simulink model "EXAMPLE_EncodeMavlink_blocks"  (R2019b)
settings: Solver=FixedStepAuto  StartTime=0.0  StopTime=inf  FixedStep=0.01  RelTol=1e-3  EnableMultiTasking=on
libraries: commutil2 x10, etargetslib x10, simulink x9, commcrc2 x5, px4uORBlib x2, px4Sensorslib x2, px4lib x1
settings Model: SimulationMode=external  ExtModeTrigDuration=10  Creator=Admin  LastModifiedBy=andrei
settings SolverCC: PositivePriorityOrder=on
settings DataIOCC: ReturnWorkspaceOutputs=off
settings OptimizationCC: EnhancedBackFolding=on  PassReuseOutputArgsAs=Individual arguments  MaxStackSize=64  OptimizeBlockOrder=speed  DifferentSizesBufferReuse=on  OptimizationCustomize=off  EfficientTunableParamExpr=on
settings DebuggingCC: ParameterTunabilityLossMsg=error  ArithmeticOperatorsInVariantConditions=warning
settings HardwareCC: ProdBitPerPointer=32  ProdBitPerSizeT=32  ProdBitPerPtrDiffT=32  ProdLargestAtomicInteger=Long  ProdLargestAtomicFloat=Double  ProdWordSize=32  ProdLongLongMode=on  ProdHWDeviceType=ARM Compatible->ARM Cortex
settings SFSimCC: SimUseLocalCustomCode=off  MATLABDynamicMemAlloc=off  CustomCodeUndefinedFunction=UseInterfaceOnly
settings RTWCC: SystemTargetFile=ert.tlc  HardwareBoard=PX4 Pixhawk 1  TLCOptions="-aInlineSetEventsForThisBaseRateFcn=TLC_FALSE -aSuppressMultiTaskScheduler=TLC_FALSE  -aRateBasedStepFcn=0"  TemplateMakefile=ert_default_tmf  GenerateReport=on  RTWUseLocalCustomCode=off  Toolchain=GNU Tools for PX4 Autopilots  IncludeHyperlinkInReport=on  LaunchReport=on  TargetLang=C++  GenerateTraceInfo=on  GenerateTraceReport=on  GenerateTraceReportSl=on  GenerateTraceReportSf=on  GenerateTraceReportEml=on
settings CodeAppCC: ForceParamTrailComments=on  IgnoreCustomStorageClasses=off  OperatorAnnotations=on  SimulinkDataObjDesc=on  SFDataObjDesc=on  InsertBlockDesc=on
settings ERTTargetCC: SupportNonInlinedSFcns=on

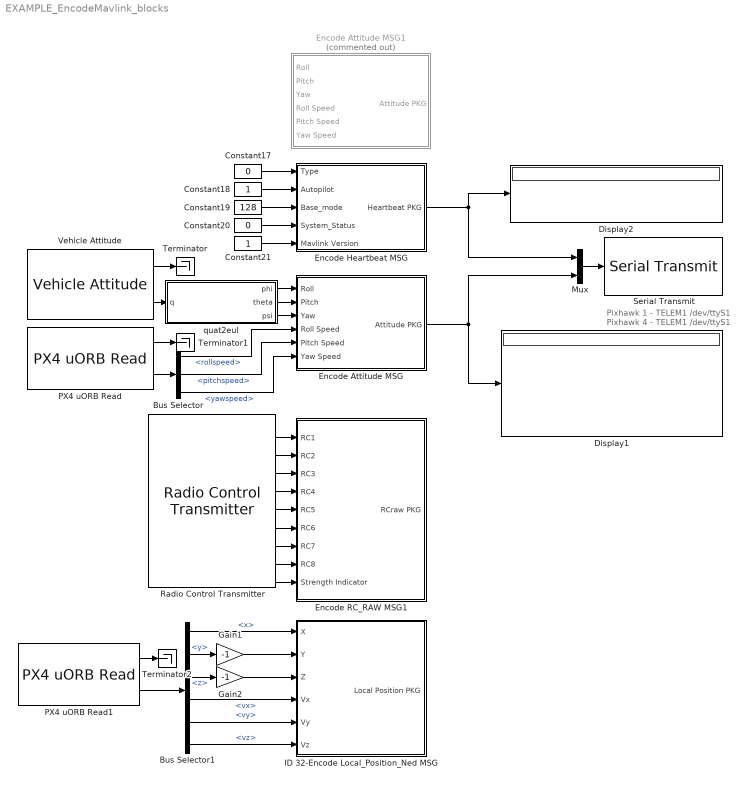
== system EXAMPLE_EncodeMavlink_blocks ==
  note: Pixhawk 1 - TELEM1 /dev/ttyS1
      | Pixhawk 4 - TELEM1 /dev/ttyS1
  Bus Selector : BusSelector  OutputSignals=rollspeed,pitchspeed,yawspeed
  Bus Selector1 : BusSelector  OutputSignals=x,y,z,vx,vy,vz
  Constant17 : Constant  Value=0
  Constant18 : Constant
  Constant19 : Constant  Value=128
  Constant20 : Constant  Value=0
  Constant21 : Constant
  Display1 : Display
  Display2 : Display
  Encode Attitude MSG : Subsystem
  Encode Attitude MSG1 : Subsystem  Commented=on
  Encode Heartbeat MSG : Subsystem
  Encode RC_RAW MSG1 : Subsystem
  Gain1 : Gain  Gain=-1
  Gain2 : Gain  Gain=-1
  ID 32-Encode Local_Position_Ned MSG : Subsystem
  Mux : Mux  Inputs=2
  PX4 uORB Read : px4uORBlib/PX4 uORB Read  uORBTopic=vehicle_attitude  sampleTime=0.01  BlockingMode=off  BlockTimeout=1e-3
      settings: SourceProductName=Embedded Coder Support Package for PX4 Autopilots  SourceProductBaseCode=PX4AUTOPILOTS
  PX4 uORB Read1 : px4uORBlib/PX4 uORB Read  uORBTopic=vehicle_local_position  sampleTime=0.01  BlockingMode=off  BlockTimeout=1e-3
      settings: SourceProductName=Embedded Coder Support Package for PX4 Autopilots  SourceProductBaseCode=PX4AUTOPILOTS
  Radio Control Transmitter : px4Sensorslib/Radio Control Transmitter  channel1=on  channel2=on  channel3=on  channel4=on  channel5=on  channel6=on  channel7=on  channel8=on  channel_count=off  rssi=on  rc_input_source=off  timestamp_last_signal=off  time_stamp=off  sampleTime=1/250  BlockingMode=off  BlockTimeout=5
      settings: SourceProductName=Embedded Coder Support Package for PX4 Autopilots
  Serial Transmit : px4lib/Serial Transmit  SCIModule=/dev/ttyS1
      settings: SourceProductName=Embedded Coder Support Package for PX4 Autopilots  SourceProductBaseCode=PX4AUTOPILOTS
  Terminator : Terminator
  Terminator1 : Terminator
  Terminator2 : Terminator
  Vehicle Attitude : px4Sensorslib/Vehicle Attitude  rollRate=off  pitchRate=off  yawRate=off  quaternion=on  uorbTimeStamp=off  BlockingMode=off  BlockTimeout=0.001  sampleTime=0.01
      settings: SourceProductName=Embedded Coder Support Package for PX4 Autopilots
  quat2eul : MATLAB Function  TreatAsAtomicUnit=on
  wires:
  Constant17/1 -> Encode Heartbeat MSG/1(Type)
  Constant18/1 -> Encode Heartbeat MSG/2(Autopilot)
  Constant19/1 -> Encode Heartbeat MSG/3(Base_mode)
  Constant20/1 -> Encode Heartbeat MSG/4(System_Status)
  Constant21/1 -> Encode Heartbeat MSG/5(Mavlink Version)
  PX4 uORB Read/1 -> Terminator1/1
  PX4 uORB Read/2 -> Bus Selector/1
  Vehicle Attitude/2 -> quat2eul/1(q)
  Vehicle Attitude/1 -> Terminator/1
  Encode Attitude MSG/1(Attitude PKG) -> Mux/2, Display1/1
  Mux/1 -> Serial Transmit/1
  Encode Heartbeat MSG/1(Heartbeat PKG) -> Mux/1, Display2/1
  quat2eul/1(phi) -> Encode Attitude MSG/1(Roll)
  quat2eul/2(theta) -> Encode Attitude MSG/2(Pitch)
  quat2eul/3(psi) -> Encode Attitude MSG/3(Yaw)
  Bus Selector/1 -> Encode Attitude MSG/4(Roll Speed)  "<rollspeed>"
  Bus Selector/2 -> Encode Attitude MSG/5(Pitch Speed)  "<pitchspeed>"
  Bus Selector/3 -> Encode Attitude MSG/6(Yaw Speed)  "<yawspeed>"
  Gain1/1 -> ID 32-Encode Local_Position_Ned MSG/2(Y)
  PX4 uORB Read1/1 -> Terminator2/1
  Gain2/1 -> ID 32-Encode Local_Position_Ned MSG/3(Z)
  Bus Selector1/4 -> ID 32-Encode Local_Position_Ned MSG/4(Vx)  "<vx>"
  Bus Selector1/5 -> ID 32-Encode Local_Position_Ned MSG/5(Vy)  "<vy>"
  PX4 uORB Read1/2 -> Bus Selector1/1
  Bus Selector1/1 -> ID 32-Encode Local_Position_Ned MSG/1(X)  "<x>"
  Bus Selector1/3 -> Gain2/1  "<z>"
  Bus Selector1/6 -> ID 32-Encode Local_Position_Ned MSG/6(Vz)  "<vz>"
  Bus Selector1/2 -> Gain1/1  "<y>"
  Radio Control Transmitter/2 -> Encode RC_RAW MSG1/1(RC1)
  Radio Control Transmitter/3 -> Encode RC_RAW MSG1/2(RC2)
  Radio Control Transmitter/4 -> Encode RC_RAW MSG1/3(RC3)
  Radio Control Transmitter/5 -> Encode RC_RAW MSG1/4(RC4)
  Radio Control Transmitter/6 -> Encode RC_RAW MSG1/5(RC5)
  Radio Control Transmitter/7 -> Encode RC_RAW MSG1/6("RC6 ")
  Radio Control Transmitter/8 -> Encode RC_RAW MSG1/7(RC7)
  Radio Control Transmitter/9 -> Encode RC_RAW MSG1/8(RC8)
  Radio Control Transmitter/10 -> Encode RC_RAW MSG1/9(Strength Indicator)

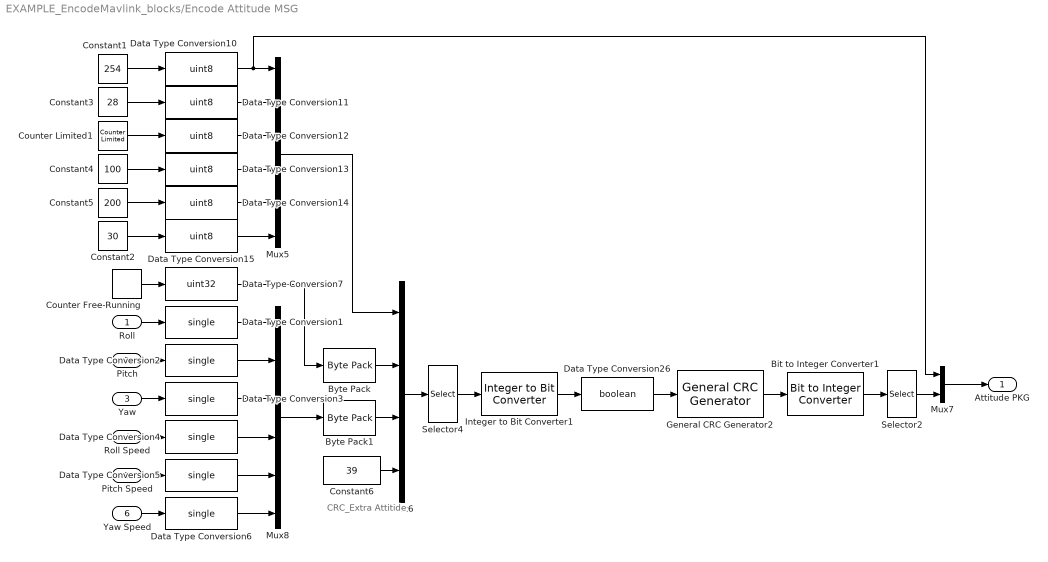
== system EXAMPLE_EncodeMavlink_blocks/Encode Attitude MSG ==
  note: CRC_Extra
      |     Attitide
  Roll : Inport
  Pitch : Inport  Port=2
  Yaw : Inport  Port=3
  Roll Speed : Inport  Port=4
  Pitch Speed : Inport  Port=5
  Yaw Speed : Inport  Port=6
  Bit to Integer Converter1 : commutil2/Bit to Integer Converter  nbits=8  bitOrder=MSB first  signedOutputValues=Unsigned  outDtype=Inherit via internal rule  outDtypeSigned=Inherit via internal rule
      settings: SourceProductName=Communications Toolbox
  Byte Pack : etargetslib/Byte Pack  datatypes={'uint32'}  byteAlign=1
      settings: SourceProductName=MATLAB Coder
  Byte Pack1 : etargetslib/Byte Pack  datatypes={'single'}  byteAlign=1
      settings: SourceProductName=MATLAB Coder
  Constant1 : Constant  Value=254
  Constant2 : Constant  Value=30
  Constant3 : Constant  Value=28
  Constant4 : Constant  Value=100
  Constant5 : Constant  Value=200
  Constant6 : Constant  Value=39  OutDataTypeStr=uint8
  Counter Free-Running : simulink/Sources/Counter Free-Running  NumBits=32  tsamp=-1
  Counter Limited1 : simulink/Sources/Counter Limited  uplimit=255  tsamp=-1
  Data Type Conversion{1..6} (6 alike) : DataTypeConversion  OutDataTypeStr=single
  Data Type Conversion{10..15} (6 alike) : DataTypeConversion  OutDataTypeStr=uint8
  Data Type Conversion26 : DataTypeConversion  OutDataTypeStr=boolean
  Data Type Conversion7 : DataTypeConversion  OutDataTypeStr=uint32
  General CRC Generator2 : commcrc2/General CRC Generator  genPoly='z^16 + z^12 + z^5 + 1'  iniStates=[1 1 1 1 1 1 1 1 1 1 1 1 1 1 1 1]  directMethod=on  reflectInputBytes=on  reflectChecksums=on  finalXOR=0  numChecksums=1
      settings: SourceProductName=Communications Toolbox  SourceProductBaseCode=CM
  Integer to Bit Converter1 : commutil2/Integer to Bit Converter  nbits=8  signedInputValues=Unsigned  bitOrder=MSB first  outDtype=Inherit via internal rule
      settings: SourceProductName=Communications Toolbox
  Mux5 : Mux  Inputs=6
  Mux6 : Mux
  Mux7 : Mux  Inputs=2
  Mux8 : Mux  Inputs=6
  Selector2 : Selector  InputPortWidth=36  IndexOptions=Index vector (dialog)  Indices=[1:33 36 35]  OutputSizes=1
  Selector4 : Selector  InputPortWidth=35  IndexOptions=Index vector (dialog)  Indices=[2:35]  OutputSizes=1
  Attitude PKG : Outport  VectorParamsAs1DForOutWhenUnconnected=off
  wires:
  Constant6/1 -> Mux6/4
  Selector4/1 -> Integer to Bit Converter1/1
  Constant1/1 -> Data Type Conversion10/1
  Constant3/1 -> Data Type Conversion11/1
  Data Type Conversion12/1 -> Mux5/3
  Data Type Conversion14/1 -> Mux5/5
  Constant4/1 -> Data Type Conversion13/1
  Data Type Conversion11/1 -> Mux5/2
  Counter Limited1/1 -> Data Type Conversion12/1
  Mux5/1 -> Mux6/1
  Yaw/1 -> Data Type Conversion3/1
  Data Type Conversion5/1 -> Mux8/5
  Data Type Conversion15/1 -> Mux5/6
  Data Type Conversion3/1 -> Mux8/3
  Mux6/1 -> Selector4/1
  Byte Pack1/1 -> Mux6/3
  Bit to Integer Converter1/1 -> Selector2/1
  Data Type Conversion2/1 -> Mux8/2
  Constant5/1 -> Data Type Conversion14/1
  Mux8/1 -> Byte Pack1/1
  Data Type Conversion7/1 -> Byte Pack/1
  Selector2/1 -> Mux7/2
  Data Type Conversion1/1 -> Mux8/1
  Yaw Speed/1 -> Data Type Conversion6/1
  Constant2/1 -> Data Type Conversion15/1
  Pitch Speed/1 -> Data Type Conversion5/1
  Data Type Conversion6/1 -> Mux8/6
  Roll/1 -> Data Type Conversion1/1
  Roll Speed/1 -> Data Type Conversion4/1
  Integer to Bit Converter1/1 -> Data Type Conversion26/1
  Data Type Conversion4/1 -> Mux8/4
  General CRC Generator2/1 -> Bit to Integer Converter1/1
  Byte Pack/1 -> Mux6/2
  Mux7/1 -> Attitude PKG/1
  Data Type Conversion13/1 -> Mux5/4
  Data Type Conversion26/1 -> General CRC Generator2/1
  Counter Free-Running/1 -> Data Type Conversion7/1
  Data Type Conversion10/1 -> Mux7/1, Mux5/1
  Pitch/1 -> Data Type Conversion2/1

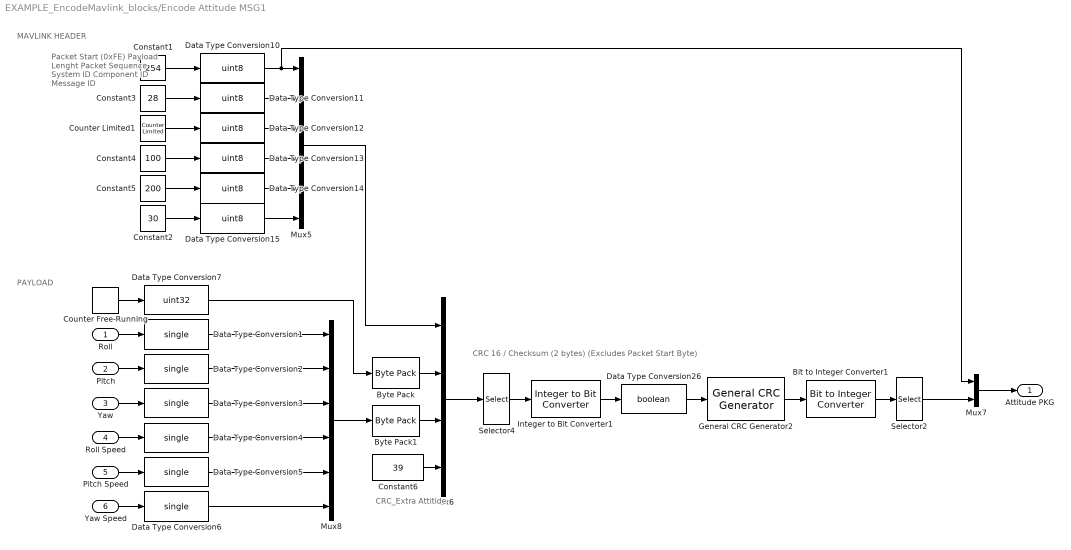
== system EXAMPLE_EncodeMavlink_blocks/Encode Attitude MSG1 ==
  note: CRC 16 / Checksum (2 bytes) (Excludes Packet Start Byte)
  note: PAYLOAD
  note: Packet Start (0xFE)
      |
      | Payload Lenght
      |
      | Packet Sequence
      |
      | System ID
      |
      | Component ID
      |
      | Message ID
  note: MAVLINK HEADER
  note: CRC_Extra
      |     Attitide
  Roll : Inport
  Pitch : Inport  Port=2
  Yaw : Inport  Port=3
  Roll Speed : Inport  Port=4
  Pitch Speed : Inport  Port=5
  Yaw Speed : Inport  Port=6
  Bit to Integer Converter1 : commutil2/Bit to Integer Converter  nbits=8  bitOrder=MSB first  signedOutputValues=Unsigned  outDtype=Inherit via internal rule  outDtypeSigned=Inherit via internal rule
      settings: SourceProductName=Communications Toolbox
  Byte Pack : etargetslib/Byte Pack  datatypes={'uint32'}  byteAlign=1
      settings: SourceProductName=MATLAB Coder
  Byte Pack1 : etargetslib/Byte Pack  datatypes={'single'}  byteAlign=1
      settings: SourceProductName=MATLAB Coder
  Constant1 : Constant  Value=254
  Constant2 : Constant  Value=30
  Constant3 : Constant  Value=28
  Constant4 : Constant  Value=100
  Constant5 : Constant  Value=200
  Constant6 : Constant  Value=39  OutDataTypeStr=uint8
  Counter Free-Running : simulink/Sources/Counter Free-Running  NumBits=32  tsamp=-1
  Counter Limited1 : simulink/Sources/Counter Limited  uplimit=7  tsamp=-1
  Data Type Conversion{1..6} (6 alike) : DataTypeConversion  OutDataTypeStr=single
  Data Type Conversion{10..15} (6 alike) : DataTypeConversion  OutDataTypeStr=uint8
  Data Type Conversion26 : DataTypeConversion  OutDataTypeStr=boolean
  Data Type Conversion7 : DataTypeConversion  OutDataTypeStr=uint32
  General CRC Generator2 : commcrc2/General CRC Generator  genPoly='z^16 + z^12 + z^5 + 1'  iniStates=[1 1 1 1 1 1 1 1 1 1 1 1 1 1 1 1]  directMethod=on  reflectInputBytes=on  reflectChecksums=on  finalXOR=0  numChecksums=1
      settings: SourceProductName=Communications Toolbox  SourceProductBaseCode=CM
  Integer to Bit Converter1 : commutil2/Integer to Bit Converter  nbits=8  signedInputValues=Unsigned  bitOrder=MSB first  outDtype=Inherit via internal rule
      settings: SourceProductName=Communications Toolbox
  Mux5 : Mux  Inputs=6
  Mux6 : Mux
  Mux7 : Mux  Inputs=2
  Mux8 : Mux  Inputs=6
  Selector2 : Selector  InputPortWidth=36  IndexOptions=Index vector (dialog)  Indices=[1:33 36 35]  OutputSizes=1
  Selector4 : Selector  InputPortWidth=35  IndexOptions=Index vector (dialog)  Indices=[2:35]  OutputSizes=1
  Attitude PKG : Outport  VectorParamsAs1DForOutWhenUnconnected=off
  wires:
  Mux7/1 -> Attitude PKG/1
  Data Type Conversion10/1 -> Mux7/1, Mux5/1
  Data Type Conversion13/1 -> Mux5/4
  Constant1/1 -> Data Type Conversion10/1
  Data Type Conversion15/1 -> Mux5/6
  Data Type Conversion12/1 -> Mux5/3
  Constant2/1 -> Data Type Conversion15/1
  Data Type Conversion11/1 -> Mux5/2
  Constant4/1 -> Data Type Conversion13/1
  Constant3/1 -> Data Type Conversion11/1
  Data Type Conversion14/1 -> Mux5/5
  Counter Limited1/1 -> Data Type Conversion12/1
  Constant5/1 -> Data Type Conversion14/1
  Mux8/1 -> Byte Pack1/1
  Counter Free-Running/1 -> Data Type Conversion7/1
  Yaw/1 -> Data Type Conversion3/1
  Byte Pack1/1 -> Mux6/3
  Roll/1 -> Data Type Conversion1/1
  Mux5/1 -> Mux6/1
  Data Type Conversion6/1 -> Mux8/6
  Byte Pack/1 -> Mux6/2
  Roll Speed/1 -> Data Type Conversion4/1
  Data Type Conversion7/1 -> Byte Pack/1
  Constant6/1 -> Mux6/4
  Data Type Conversion2/1 -> Mux8/2
  Data Type Conversion3/1 -> Mux8/3
  Data Type Conversion5/1 -> Mux8/5
  Pitch Speed/1 -> Data Type Conversion5/1
  Yaw Speed/1 -> Data Type Conversion6/1
  Data Type Conversion1/1 -> Mux8/1
  Data Type Conversion4/1 -> Mux8/4
  Pitch/1 -> Data Type Conversion2/1
  Selector2/1 -> Mux7/2
  Mux6/1 -> Selector4/1
  General CRC Generator2/1 -> Bit to Integer Converter1/1
  Bit to Integer Converter1/1 -> Selector2/1
  Integer to Bit Converter1/1 -> Data Type Conversion26/1
  Selector4/1 -> Integer to Bit Converter1/1
  Data Type Conversion26/1 -> General CRC Generator2/1

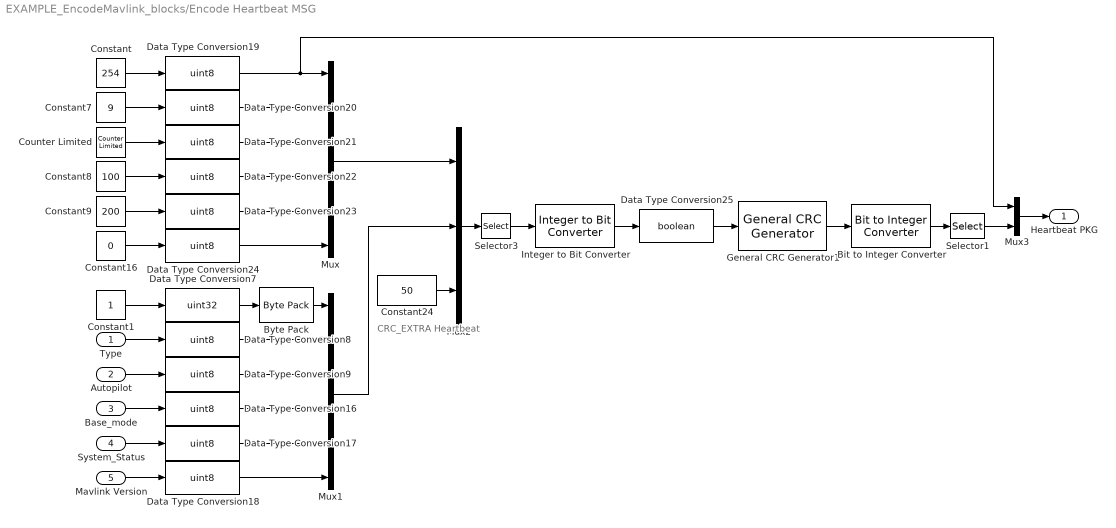
== system EXAMPLE_EncodeMavlink_blocks/Encode Heartbeat MSG ==
  note: CRC_EXTRA
      |    Heartbeat
  Type : Inport
  Autopilot : Inport  Port=2
  Base_mode : Inport  Port=3
  System_Status : Inport  Port=4
  Mavlink Version : Inport  Port=5
  Bit to Integer Converter : commutil2/Bit to Integer Converter  nbits=8  bitOrder=MSB first  signedOutputValues=Unsigned  outDtype=Inherit via internal rule  outDtypeSigned=Inherit via internal rule
      settings: SourceProductName=Communications Toolbox
  Byte Pack : etargetslib/Byte Pack  datatypes={'uint32'}  byteAlign=1
      settings: SourceProductName=MATLAB Coder
  Constant : Constant  Value=254
  Constant1 : Constant
  Constant16 : Constant  Value=0
  Constant24 : Constant  Value=50  OutDataTypeStr=uint8
  Constant7 : Constant  Value=9
  Constant8 : Constant  Value=100
  Constant9 : Constant  Value=200
  Counter Limited : simulink/Sources/Counter Limited  uplimit=255  tsamp=-1
  Data Type Conversion{8..9,16..24} (11 alike) : DataTypeConversion  OutDataTypeStr=uint8
  Data Type Conversion25 : DataTypeConversion  OutDataTypeStr=boolean
  Data Type Conversion7 : DataTypeConversion  OutDataTypeStr=uint32
  General CRC Generator1 : commcrc2/General CRC Generator  genPoly='z^16 + z^12 + z^5 + 1'  iniStates=[1 1 1 1 1 1 1 1 1 1 1 1 1 1 1 1]  directMethod=on  reflectInputBytes=on  reflectChecksums=on  finalXOR=0  numChecksums=1
      settings: SourceProductName=Communications Toolbox  SourceProductBaseCode=CM
  Integer to Bit Converter : commutil2/Integer to Bit Converter  nbits=8  signedInputValues=Unsigned  bitOrder=MSB first  outDtype=Inherit via internal rule
      settings: SourceProductName=Communications Toolbox
  Mux : Mux  Inputs=6
  Mux1 : Mux  Inputs=6
  Mux2 : Mux  Inputs=3
  Mux3 : Mux  Inputs=2
  Selector1 : Selector  InputPortWidth=17  IndexOptions=Index vector (dialog)  Indices=[1:14 17 16]  OutputSizes=1
  Selector3 : Selector  InputPortWidth=16  IndexOptions=Index vector (dialog)  Indices=[2:16]  OutputSizes=1
  Heartbeat PKG : Outport  VectorParamsAs1DForOutWhenUnconnected=off
  wires:
  Data Type Conversion23/1 -> Mux/5
  Data Type Conversion8/1 -> Mux1/2
  Constant9/1 -> Data Type Conversion23/1
  Data Type Conversion24/1 -> Mux/6
  Constant24/1 -> Mux2/3
  Byte Pack/1 -> Mux1/1
  Data Type Conversion9/1 -> Mux1/3
  Mux/1 -> Mux2/1
  Integer to Bit Converter/1 -> Data Type Conversion25/1
  Bit to Integer Converter/1 -> Selector1/1
  Mux2/1 -> Selector3/1
  Selector3/1 -> Integer to Bit Converter/1
  Data Type Conversion19/1 -> Mux3/1, Mux/1
  Mux3/1 -> Heartbeat PKG/1
  Base_mode/1 -> Data Type Conversion16/1
  Autopilot/1 -> Data Type Conversion9/1
  Data Type Conversion20/1 -> Mux/2
  Mux1/1 -> Mux2/2
  Type/1 -> Data Type Conversion8/1
  Data Type Conversion7/1 -> Byte Pack/1
  Constant/1 -> Data Type Conversion19/1
  Data Type Conversion22/1 -> Mux/4
  Data Type Conversion16/1 -> Mux1/4
  System_Status/1 -> Data Type Conversion17/1
  General CRC Generator1/1 -> Bit to Integer Converter/1
  Data Type Conversion25/1 -> General CRC Generator1/1
  Data Type Conversion17/1 -> Mux1/5
  Mavlink Version/1 -> Data Type Conversion18/1
  Constant1/1 -> Data Type Conversion7/1
  Selector1/1 -> Mux3/2
  Data Type Conversion21/1 -> Mux/3
  Counter Limited/1 -> Data Type Conversion21/1
  Data Type Conversion18/1 -> Mux1/6
  Constant8/1 -> Data Type Conversion22/1
  Constant7/1 -> Data Type Conversion20/1
  Constant16/1 -> Data Type Conversion24/1

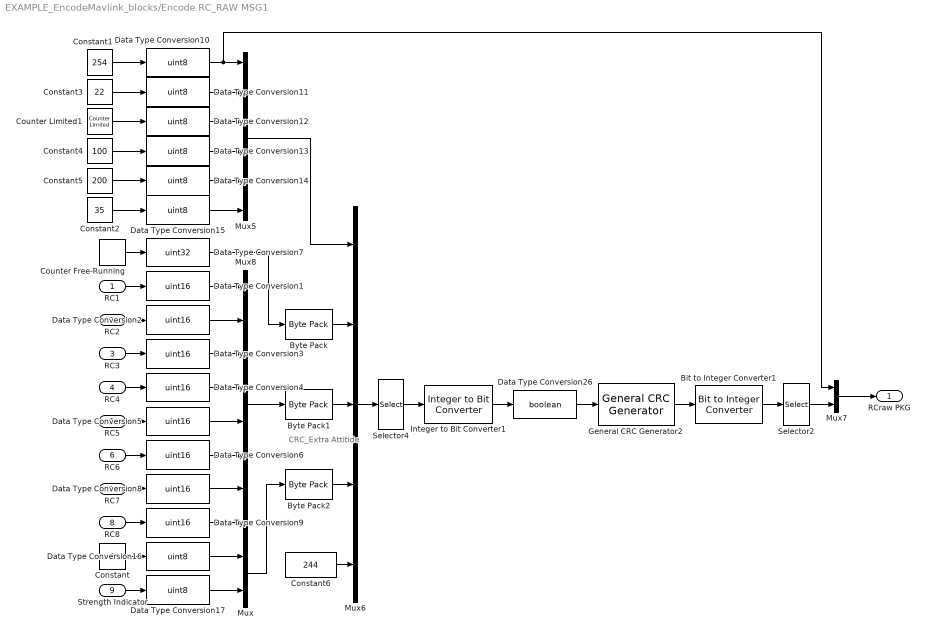
== system EXAMPLE_EncodeMavlink_blocks/Encode RC_RAW MSG1 ==
  note: CRC_Extra
      |     Attitide
  RC1 : Inport
  RC2 : Inport  Port=2
  RC3 : Inport  Port=3
  RC4 : Inport  Port=4
  RC5 : Inport  Port=5
  "RC6 " : Inport  Port=6
  RC7 : Inport  Port=7
  RC8 : Inport  Port=8
  Strength Indicator : Inport  Port=9
  Bit to Integer Converter1 : commutil2/Bit to Integer Converter  nbits=8  bitOrder=MSB first  signedOutputValues=Unsigned  outDtype=Inherit via internal rule  outDtypeSigned=Inherit via internal rule
      settings: SourceProductName=Communications Toolbox
  Byte Pack : etargetslib/Byte Pack  datatypes={'uint32'}  byteAlign=1
      settings: SourceProductName=MATLAB Coder
  Byte Pack1 : etargetslib/Byte Pack  datatypes={'uint16'}  byteAlign=1
      settings: SourceProductName=MATLAB Coder
  Byte Pack2 : etargetslib/Byte Pack  datatypes={'uint8'}  byteAlign=1
      settings: SourceProductName=MATLAB Coder
  Constant : Constant  Value=0
  Constant1 : Constant  Value=254
  Constant2 : Constant  Value=35
  Constant3 : Constant  Value=22
  Constant4 : Constant  Value=100
  Constant5 : Constant  Value=200
  Constant6 : Constant  Value=244  OutDataTypeStr=uint8
  Counter Free-Running : simulink/Sources/Counter Free-Running  NumBits=32  tsamp=-1
  Counter Limited1 : simulink/Sources/Counter Limited  uplimit=255  tsamp=-1
  Data Type Conversion{1..6,8..9} (8 alike) : DataTypeConversion  OutDataTypeStr=uint16
  Data Type Conversion{10..17} (8 alike) : DataTypeConversion  OutDataTypeStr=uint8
  Data Type Conversion26 : DataTypeConversion  OutDataTypeStr=boolean
  Data Type Conversion7 : DataTypeConversion  OutDataTypeStr=uint32
  General CRC Generator2 : commcrc2/General CRC Generator  genPoly='z^16 + z^12 + z^5 + 1'  iniStates=[1 1 1 1 1 1 1 1 1 1 1 1 1 1 1 1]  directMethod=on  reflectInputBytes=on  reflectChecksums=on  finalXOR=0  numChecksums=1
      settings: SourceProductName=Communications Toolbox  SourceProductBaseCode=CM
  Integer to Bit Converter1 : commutil2/Integer to Bit Converter  nbits=8  signedInputValues=Unsigned  bitOrder=MSB first  outDtype=Inherit via internal rule
      settings: SourceProductName=Communications Toolbox
  Mux : Mux  Inputs=2
  Mux5 : Mux  Inputs=6
  Mux6 : Mux  Inputs=5
  Mux7 : Mux  Inputs=2
  Mux8 : Mux  Inputs=8
  Selector2 : Selector  InputPortWidth=30  IndexOptions=Index vector (dialog)  Indices=[1:28 30 29]  OutputSizes=1
  Selector4 : Selector  InputPortWidth=29  IndexOptions=Index vector (dialog)  Indices=[2:29]  OutputSizes=1
  RCraw PKG : Outport  VectorParamsAs1DForOutWhenUnconnected=off
  wires:
  Selector4/1 -> Integer to Bit Converter1/1
  Constant1/1 -> Data Type Conversion10/1
  Constant3/1 -> Data Type Conversion11/1
  Data Type Conversion12/1 -> Mux5/3
  Data Type Conversion14/1 -> Mux5/5
  Constant4/1 -> Data Type Conversion13/1
  Data Type Conversion11/1 -> Mux5/2
  Counter Limited1/1 -> Data Type Conversion12/1
  Mux5/1 -> Mux6/1
  RC3/1 -> Data Type Conversion3/1
  Data Type Conversion15/1 -> Mux5/6
  Mux6/1 -> Selector4/1
  Byte Pack1/1 -> Mux6/3
  Bit to Integer Converter1/1 -> Selector2/1
  Constant5/1 -> Data Type Conversion14/1
  Mux8/1 -> Byte Pack1/1
  Data Type Conversion7/1 -> Byte Pack/1
  Selector2/1 -> Mux7/2
  "RC6 "/1 -> Data Type Conversion6/1
  Constant2/1 -> Data Type Conversion15/1
  RC5/1 -> Data Type Conversion5/1
  RC1/1 -> Data Type Conversion1/1
  RC4/1 -> Data Type Conversion4/1
  Integer to Bit Converter1/1 -> Data Type Conversion26/1
  General CRC Generator2/1 -> Bit to Integer Converter1/1
  Byte Pack/1 -> Mux6/2
  Mux7/1 -> RCraw PKG/1
  Data Type Conversion13/1 -> Mux5/4
  Data Type Conversion26/1 -> General CRC Generator2/1
  Counter Free-Running/1 -> Data Type Conversion7/1
  Data Type Conversion10/1 -> Mux7/1, Mux5/1
  RC2/1 -> Data Type Conversion2/1
  Data Type Conversion1/1 -> Mux8/1
  Data Type Conversion2/1 -> Mux8/2
  Data Type Conversion3/1 -> Mux8/3
  Data Type Conversion4/1 -> Mux8/4
  Data Type Conversion5/1 -> Mux8/5
  Data Type Conversion6/1 -> Mux8/6
  Data Type Conversion8/1 -> Mux8/7
  Data Type Conversion9/1 -> Mux8/8
  RC7/1 -> Data Type Conversion8/1
  RC8/1 -> Data Type Conversion9/1
  Strength Indicator/1 -> Data Type Conversion17/1
  Constant/1 -> Data Type Conversion16/1
  Data Type Conversion16/1 -> Mux/1
  Data Type Conversion17/1 -> Mux/2
  Mux/1 -> Byte Pack2/1
  Byte Pack2/1 -> Mux6/4
  Constant6/1 -> Mux6/5

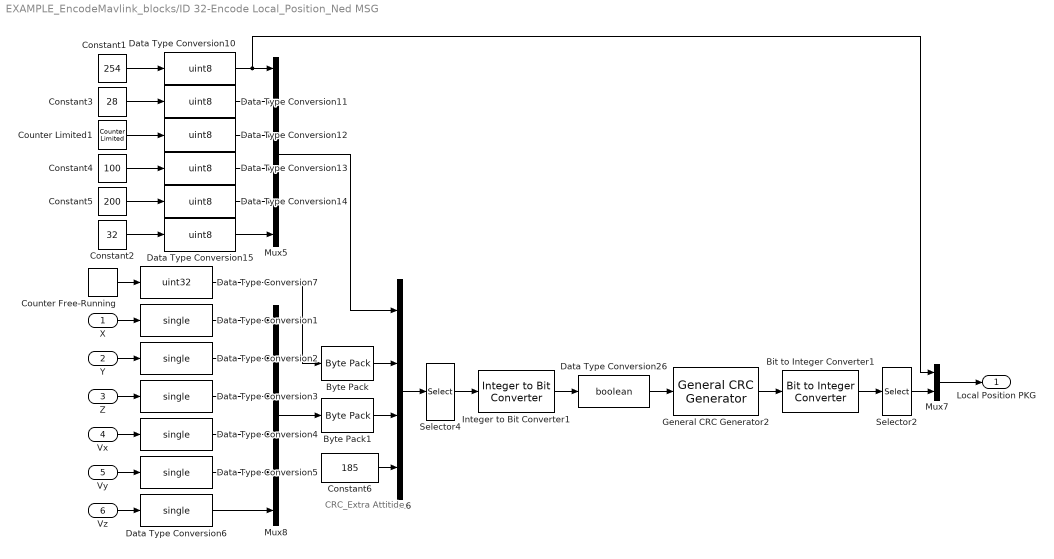
== system EXAMPLE_EncodeMavlink_blocks/ID 32-Encode Local_Position_Ned MSG ==
  note: CRC_Extra
      |     Attitide
  X : Inport
  Y : Inport  Port=2
  Z : Inport  Port=3
  Vx : Inport  Port=4
  Vy : Inport  Port=5
  Vz : Inport  Port=6
  Bit to Integer Converter1 : commutil2/Bit to Integer Converter  nbits=8  bitOrder=MSB first  signedOutputValues=Unsigned  outDtype=Inherit via internal rule  outDtypeSigned=Inherit via internal rule
      settings: SourceProductName=Communications Toolbox
  Byte Pack : etargetslib/Byte Pack  datatypes={'uint32'}  byteAlign=1
      settings: SourceProductName=MATLAB Coder
  Byte Pack1 : etargetslib/Byte Pack  datatypes={'single'}  byteAlign=1
      settings: SourceProductName=MATLAB Coder
  Constant1 : Constant  Value=254
  Constant2 : Constant  Value=32
  Constant3 : Constant  Value=28
  Constant4 : Constant  Value=100
  Constant5 : Constant  Value=200
  Constant6 : Constant  Value=185  OutDataTypeStr=uint8
  Counter Free-Running : simulink/Sources/Counter Free-Running  NumBits=32  tsamp=-1
  Counter Limited1 : simulink/Sources/Counter Limited  uplimit=255  tsamp=-1
  Data Type Conversion{1..6} (6 alike) : DataTypeConversion  OutDataTypeStr=single
  Data Type Conversion{10..15} (6 alike) : DataTypeConversion  OutDataTypeStr=uint8
  Data Type Conversion26 : DataTypeConversion  OutDataTypeStr=boolean
  Data Type Conversion7 : DataTypeConversion  OutDataTypeStr=uint32
  General CRC Generator2 : commcrc2/General CRC Generator  genPoly='z^16 + z^12 + z^5 + 1'  iniStates=[1 1 1 1 1 1 1 1 1 1 1 1 1 1 1 1]  directMethod=on  reflectInputBytes=on  reflectChecksums=on  finalXOR=0  numChecksums=1
      settings: SourceProductName=Communications Toolbox  SourceProductBaseCode=CM
  Integer to Bit Converter1 : commutil2/Integer to Bit Converter  nbits=8  signedInputValues=Unsigned  bitOrder=MSB first  outDtype=Inherit via internal rule
      settings: SourceProductName=Communications Toolbox
  Mux5 : Mux  Inputs=6
  Mux6 : Mux
  Mux7 : Mux  Inputs=2
  Mux8 : Mux  Inputs=6
  Selector2 : Selector  InputPortWidth=36  IndexOptions=Index vector (dialog)  Indices=[1:33 36 35]  OutputSizes=1
  Selector4 : Selector  InputPortWidth=35  IndexOptions=Index vector (dialog)  Indices=[2:35]  OutputSizes=1
  Local Position PKG : Outport  VectorParamsAs1DForOutWhenUnconnected=off
  wires:
  Constant6/1 -> Mux6/4
  Selector4/1 -> Integer to Bit Converter1/1
  Constant1/1 -> Data Type Conversion10/1
  Constant3/1 -> Data Type Conversion11/1
  Data Type Conversion12/1 -> Mux5/3
  Data Type Conversion14/1 -> Mux5/5
  Constant4/1 -> Data Type Conversion13/1
  Data Type Conversion11/1 -> Mux5/2
  Counter Limited1/1 -> Data Type Conversion12/1
  Mux5/1 -> Mux6/1
  Z/1 -> Data Type Conversion3/1
  Data Type Conversion5/1 -> Mux8/5
  Data Type Conversion15/1 -> Mux5/6
  Data Type Conversion3/1 -> Mux8/3
  Mux6/1 -> Selector4/1
  Byte Pack1/1 -> Mux6/3
  Bit to Integer Converter1/1 -> Selector2/1
  Data Type Conversion2/1 -> Mux8/2
  Constant5/1 -> Data Type Conversion14/1
  Mux8/1 -> Byte Pack1/1
  Data Type Conversion7/1 -> Byte Pack/1
  Selector2/1 -> Mux7/2
  Data Type Conversion1/1 -> Mux8/1
  Vz/1 -> Data Type Conversion6/1
  Constant2/1 -> Data Type Conversion15/1
  Vy/1 -> Data Type Conversion5/1
  X/1 -> Data Type Conversion1/1
  Vx/1 -> Data Type Conversion4/1
  Integer to Bit Converter1/1 -> Data Type Conversion26/1
  Data Type Conversion4/1 -> Mux8/4
  General CRC Generator2/1 -> Bit to Integer Converter1/1
  Byte Pack/1 -> Mux6/2
  Mux7/1 -> Local Position PKG/1
  Data Type Conversion13/1 -> Mux5/4
  Data Type Conversion26/1 -> General CRC Generator2/1
  Counter Free-Running/1 -> Data Type Conversion7/1
  Data Type Conversion10/1 -> Mux7/1, Mux5/1
  Y/1 -> Data Type Conversion2/1
  Data Type Conversion6/1 -> Mux8/6

== matlab function EXAMPLE_EncodeMavlink_blocks/quat2eul ==
  data: q input; phi output; theta output; psi output
function [phi,theta,psi] = quat2eul(q)

% Quaternion conversion to Euler angles based on the PX4 Firmware v1.6.5
% release.

phi = atan2(2*(q(1)*q(2) + q(3)* q(4)), q(1)^2 - q(2)^2 - q(3)^2 + q(4)^2);
theta = asin(-2*(q(2)*q(4) - q(1)*q(3)));
psi = atan2(2*(q(2)*q(3) + q(1)* q(4)), q(1)^2 + q(2)^2 - q(3)^2 - q(4)^2);

end
